simulink model "Switching_logic_block"  (R2021a)
settings: Solver=VariableStepAuto  StartTime=0.0  StopTime=10.0  RelTol=1e-3
settings Model: Creator=wwwvi  LastModifiedBy=wwwvi

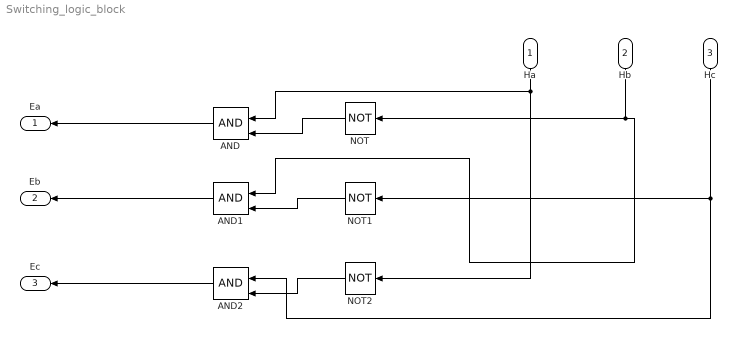
== system Switching_logic_block ==
  Ha : Inport
  Hb : Inport  Port=2
  Hc : Inport  Port=3
  AND : Logic  IconShape=distinctive  AllPortsSameDT=off  OutDataTypeStr=boolean
  AND1 : Logic  IconShape=distinctive  AllPortsSameDT=off  OutDataTypeStr=boolean
  AND2 : Logic  IconShape=distinctive  AllPortsSameDT=off  OutDataTypeStr=boolean
  NOT : Logic  Operator=NOT  IconShape=distinctive  AllPortsSameDT=off  OutDataTypeStr=boolean
  NOT1 : Logic  Operator=NOT  IconShape=distinctive  AllPortsSameDT=off  OutDataTypeStr=boolean
  NOT2 : Logic  Operator=NOT  IconShape=distinctive  AllPortsSameDT=off  OutDataTypeStr=boolean
  Ea : Outport
  Eb : Outport  Port=2
  Ec : Outport  Port=3
  wires:
  NOT/1 -> AND/2
  NOT1/1 -> AND1/2
  NOT2/1 -> AND2/2
  Ha/1 -> AND/1, NOT2/1
  Hb/1 -> AND1/1, NOT/1
  AND/1 -> Ea/1
  AND1/1 -> Eb/1
  AND2/1 -> Ec/1
  Hc/1 -> NOT1/1, AND2/1
